simulink model "ImproveMotorIdent"  (R2013a)
settings: Solver=FixedStepDiscrete  StartTime=0.0  StopTime=Time  FixedStep=0.01  RelTol=1e-3
values from neighbouring files (symbols this model uses):
  joint = CoupledJoints('experiments', 'iCubGenova03', 'torso')    [CoupledExper-IDLE.m]    (also in CoupledExper.m = joint.loadRefFile('ref'); CoupledJoints.m = [joint Motor(date,robotName, part, type,'yaw')]; FrictionTest.m = joint.loadFriction('idle.mat',1); JointStructure.m = struct)
  Reference = struct    [CoupledJoints.m]    (also in ReferenceLoad.m; WBLMotor.m)
libraries: WBCLibrary x19, utility x1
settings Model: Creator=Raffaello  LastModifiedBy=Raffaello
settings DataIOCC: LimitDataPoints=off  OutputSaveName=out

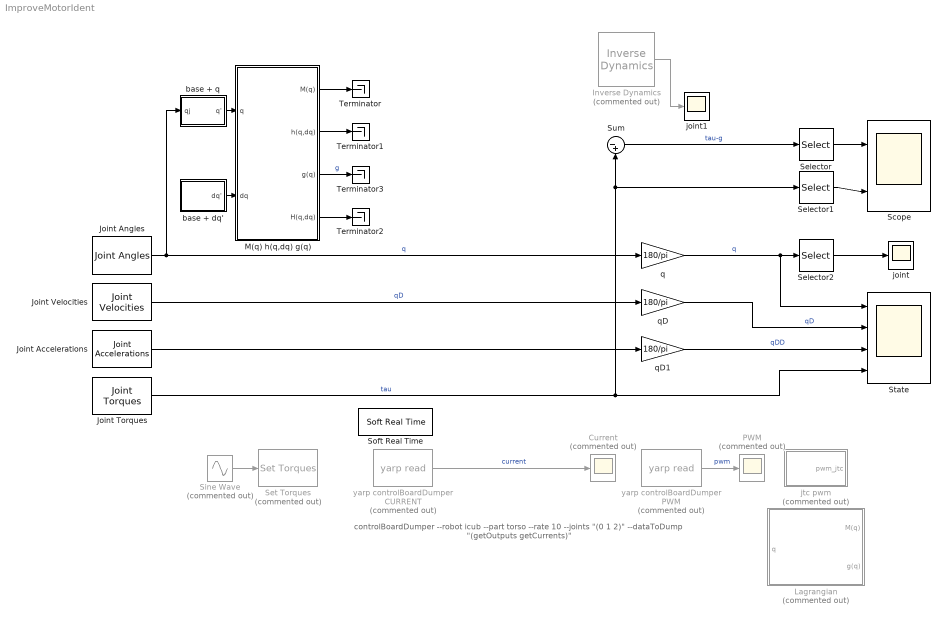
== system ImproveMotorIdent ==
  note: controlBoardDumper --robot icub --part torso --rate 10 --joints "(0 1 2)" --dataToDump "(getOutputs getCurrents)"
  Current : Scope  Commented=on
      settings: YMin=-3750  YMax=1750  SaveName=ScopeData3
  Inverse Dynamics : WBCLibrary/wholeBodyModel/Dynamics/Inverse Dynamics  Commented=on  robotName=robotName  localName=localName
  Joint Accelerations : WBCLibrary/wholeBodyStates/Joint Accelerations  robotName=robotName  localName=localName
  Joint Angles : WBCLibrary/wholeBodyStates/Joint Angles  robotName=robotName  localName=localName
  Joint Torques : WBCLibrary/wholeBodyStates/Joint Torques  robotName=robotName  localName=localName
  Joint Velocities : WBCLibrary/wholeBodyStates/Joint Velocities  robotName=robotName  localName=localName
  Lagrangian : Subsystem  Commented=on
  M(q) h(q,dq) g(q) : Subsystem
  PWM : Scope  Commented=on
      settings: YMin=260  YMax=295
  Scope : Scope  NumInputPorts=2
      settings: TimeRange=60  YMin=-1.5~-1.5  YMax=2~2  SaveName=ScopeData5
  Selector : Selector  InputPortWidth=25  IndexOptions=Index vector (dialog)  Indices=[joint.number]  OutputSizes=1
  Selector1 : Selector  InputPortWidth=25  IndexOptions=Index vector (dialog)  Indices=[joint.number]  OutputSizes=1
  Selector2 : Selector  InputPortWidth=25  IndexOptions=Index vector (dialog)  Indices=[joint.number]  OutputSizes=1
  Set Torques : WBCLibrary/wholeBodyActuators/Set Torques  Commented=on  val=6  robotName=robotName  localName=localName
  Sine Wave : Sin  Commented=on  Amplitude=Reference.sinAmp  Bias=Reference.sinBias  Frequency=Reference.sinFreq*2*pi  SampleTime=0
  Soft Real Time : utility/Soft Real Time  x=1
  State : Scope  NumInputPorts=4
      settings: TimeRange=60  YMin=-100~-0.5~-8~-2.5  YMax=125~0.5~5~2  SaveName=ScopeData2
  Sum : Sum  Inputs=|-+
  Terminator{,1..3} (4 alike) : Terminator
  base + dq' : Subsystem
  base + q : Subsystem
  joint : Scope
      settings: YMin=63.022  YMax=63.022  SaveName=ScopeData4
  joint1 : Scope
      settings: YMin=0  YMax=19  SaveName=ScopeData6
  jtc pwm : Subsystem  Commented=on
  q : Gain  Gain=180/pi
  qD : Gain  Gain=180/pi
  qD1 : Gain  Gain=180/pi
  yarp controlBoardDumper CURRENT : WBCLibrary/Utilities/yarp read  Commented=on  from=['/controlBoardDumper/' joint.path '/getCurrents']  to='...'  num=1  blocking=off  timestamp=off
  yarp controlBoardDumper PWM : WBCLibrary/Utilities/yarp read  Commented=on  from=['/controlBoardDumper/' joint.path '/getOutputs']  to='...'  num=1  blocking=off  timestamp=off
  wires:
  Sine Wave/1 -> Set Torques/1
  Joint Angles/1 -> q/1, base + q/1(qj)  "q"
  Joint Velocities/1 -> qD/1  "qD"
  Joint Torques/1 -> Selector1/1, Sum/2, State/4  "tau"
  q/1 -> Selector2/1, State/1  "q"
  qD/1 -> State/2  "qD"
  yarp controlBoardDumper PWM/1 -> PWM/1  "pwm"
  yarp controlBoardDumper CURRENT/1 -> Current/1  "current"
  Joint Accelerations/1 -> qD1/1
  qD1/1 -> State/3  "qDD"
  Sum/1 -> Selector/1  "tau-g"
  M(q) h(q,dq) g(q)/3(g(q)) -> Terminator3/1  "g"
  Selector/1 -> Scope/1
  Selector1/1 -> Scope/2
  Selector2/1 -> joint/1
  Inverse Dynamics/1 -> joint1/1
  base + q/1(q') -> M(q) h(q,dq) g(q)/1(q)
  base + dq'/1(dq') -> M(q) h(q,dq) g(q)/2(dq)
  M(q) h(q,dq) g(q)/1(M(q)) -> Terminator/1
  M(q) h(q,dq) g(q)/2(h(q,dq)) -> Terminator1/1
  M(q) h(q,dq) g(q)/4(H(q,dq)) -> Terminator2/1

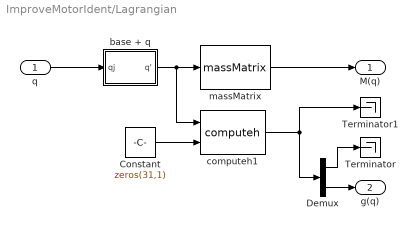
== system ImproveMotorIdent/Lagrangian ==
  q : Inport
  Constant : Constant  Value=zeros(31,1)
  Demux : Demux  Outputs=[6, 25]
  Terminator : Terminator
  Terminator1 : Terminator
  base + q : Subsystem
  computeh1 : WBCLibrary/wholeBodyModel/Dynamics/computeh  val=7  robotname=robotName  localname=localName
  massMatrix : WBCLibrary/wholeBodyModel/Dynamics/massMatrix  val=8  robotname=robotName  localname=localName
  M(q) : Outport
  g(q) : Outport  Port=2
  wires:
  q/1 -> base + q/1(qj)
  Constant/1 -> computeh1/2
  base + q/1(q') -> massMatrix/1, computeh1/1
  computeh1/1 -> Terminator1/1, Demux/1
  massMatrix/1 -> M(q)/1
  Demux/1 -> Terminator/1
  Demux/2 -> g(q)/1

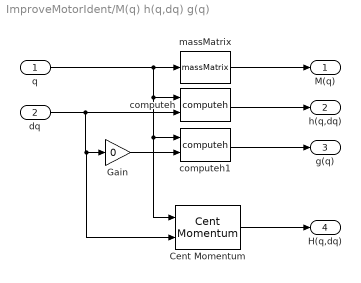
== system ImproveMotorIdent/M(q) h(q,dq) g(q) ==
  q : Inport
  dq : Inport  Port=2
  Cent Momentum : WBCLibrary/wholeBodyModel/Dynamics/Cent Momentum  robotName=robotName  localName=localName
  Gain : Gain  Gain=0
  computeh : WBCLibrary/wholeBodyModel/Dynamics/computeh  val=7  robotname=robotName  localname=localName
  computeh1 : WBCLibrary/wholeBodyModel/Dynamics/computeh  val=7  robotname=robotName  localname=localName
  massMatrix : WBCLibrary/wholeBodyModel/Dynamics/massMatrix  val=8  robotname=robotName  localname=localName
  M(q) : Outport
  h(q,dq) : Outport  Port=2
  g(q) : Outport  Port=3
  H(q,dq) : Outport  Port=4
  wires:
  Gain/1 -> computeh1/2
  computeh1/1 -> g(q)/1
  computeh/1 -> h(q,dq)/1
  massMatrix/1 -> M(q)/1
  q/1 -> Cent Momentum/1, computeh1/1, computeh/1, massMatrix/1
  dq/1 -> Cent Momentum/2, Gain/1, computeh/2
  Cent Momentum/1 -> H(q,dq)/1

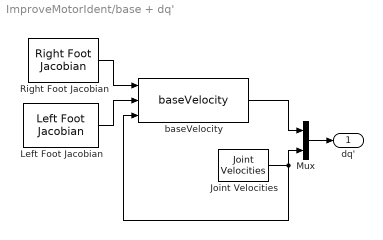
== system ImproveMotorIdent/base + dq' ==
  Joint Velocities : WBCLibrary/wholeBodyStates/Joint Velocities  robotName=robotName  localName=localName
  Left Foot Jacobian : WBCLibrary/wholeBodyModel/Jacobians/Left Foot Jacobian  robotName=robotName  localName=localName
  Mux : Mux  Inputs=2
  Right Foot Jacobian : WBCLibrary/wholeBodyModel/Jacobians/Right Foot Jacobian  robotName=robotName  localName=localName
  baseVelocity : WBCLibrary/Utilities/baseVelocity
  dq' : Outport
  wires:
  Left Foot Jacobian/1 -> baseVelocity/2
  Right Foot Jacobian/1 -> baseVelocity/1
  baseVelocity/1 -> Mux/1
  Joint Velocities/1 -> baseVelocity/3, Mux/2
  Mux/1 -> dq'/1

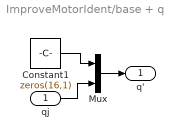
== system ImproveMotorIdent/base + q ==
  qj : Inport
  Constant1 : Constant  Value=zeros(16,1)
  Mux : Mux  Inputs=2
  q' : Outport
  wires:
  Mux/1 -> q'/1
  qj/1 -> Mux/2
  Constant1/1 -> Mux/1

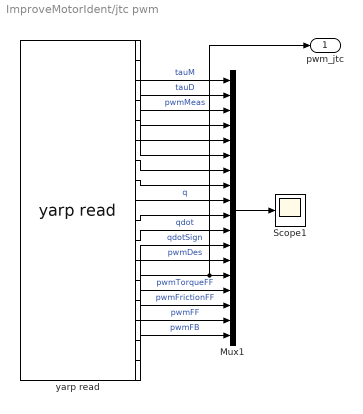
== system ImproveMotorIdent/jtc pwm ==
  Mux1 : Mux  Inputs=18
  Scope1 : Scope
      settings: ShowLegends=on
  yarp read : WBCLibrary/Utilities/yarp read  from=['/jtc/monitor:o']  to='...'  num=18  blocking=off  timestamp=off
  pwm_jtc : Outport
  wires:
  yarp read/18 -> Mux1/18  "pwmFB"
  Mux1/1 -> Scope1/1
  yarp read/1 -> Mux1/1  "tauM"
  yarp read/2 -> Mux1/2  "tauD"
  yarp read/3 -> Mux1/3
  yarp read/4 -> Mux1/4
  yarp read/5 -> Mux1/5
  yarp read/10 -> Mux1/10
  yarp read/6 -> Mux1/6
  yarp read/7 -> Mux1/7
  yarp read/8 -> Mux1/8
  yarp read/9 -> Mux1/9  "q"
  yarp read/11 -> Mux1/11  "qdot"
  yarp read/12 -> Mux1/12  "qdotSign"
  yarp read/13 -> Mux1/13  "pwmDes"
  yarp read/14 -> pwm_jtc/1, Mux1/14  "pwmMeas"
  yarp read/15 -> Mux1/15  "pwmTorqueFF"
  yarp read/16 -> Mux1/16  "pwmFrictionFF"
  yarp read/17 -> Mux1/17  "pwmFF"

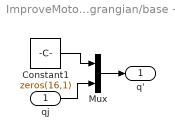
== system ImproveMotorIdent/Lagrangian/base + q ==
  qj : Inport
  Constant1 : Constant  Value=zeros(16,1)
  Mux : Mux  Inputs=2
  q' : Outport
  wires:
  Mux/1 -> q'/1
  qj/1 -> Mux/2
  Constant1/1 -> Mux/1
